simulink model "MotorCtrl_DTC_Math"  (R2023b)
settings: Solver=FixedStepDiscrete  StartTime=0.0  StopTime=5  FixedStep=MC_Sim_BaseStep  RelTol=1e-3  EnableMultiTasking=on
values from neighbouring files (symbols this model uses):
  MC_ADC_BitNum = 0.0    [MotorControlDataDictionary_Math.sldd]
  MC_ADC_Offset = 0.0    [MotorControlDataDictionary_Math.sldd]
  MC_ADC_VRef = 1.0    [MotorControlDataDictionary_Math.sldd]
  MC_Const_DutyL = 0.2    [MotorControlDataDictionary_Math.sldd]
  MC_Const_DutyS = 0.8    [MotorControlDataDictionary_Math.sldd]
  MC_CSA_Gain = 1.0    [MotorControlDataDictionary_Math.sldd]
  MC_Input_Vdc = 13.5    [MotorControlDataDictionary_Math.sldd]
  MC_MOS_DeadTime = 1.0E-6    [MotorControlDataDictionary_Math.sldd]
  MC_Motor_Mechinal_Damp = 1.0E-5    [MotorControlDataDictionary_Math.sldd]
  MC_Motor_Mechinal_Fric = 0.0    [MotorControlDataDictionary_Math.sldd]
  MC_Motor_Mechinal_Inertia = 0.0103    [MotorControlDataDictionary_Math.sldd]
  MC_Motor_Phi = 0.0059190254913385806    [MotorControlDataDictionary_Math.sldd]
  MC_Motor_Rotor_Pn = 4.0    [MotorControlDataDictionary_Math.sldd]
  MC_Motor_Stator_Ld = 5.6345E-5    [MotorControlDataDictionary_Math.sldd]
  MC_Motor_Stator_Lq = 5.6345E-5    [MotorControlDataDictionary_Math.sldd]
  MC_Motor_Stator_Rs = 0.0286    [MotorControlDataDictionary_Math.sldd]
  MC_Param_CurrentPI_Ki = 0.0071879639914134473    [MotorControlDataDictionary_Math.sldd]
  MC_Param_CurrentPI_Kp = 0.283220860906427    [MotorControlDataDictionary_Math.sldd]
  MC_Param_CurrentPI_UdInteMax = 7.794228634059948    [MotorControlDataDictionary_Math.sldd]
  MC_Param_CurrentPI_UdInteMin = -7.794228634059948    [MotorControlDataDictionary_Math.sldd]
  MC_Param_CurrentPI_UdMax = 7.794228634059948    [MotorControlDataDictionary_Math.sldd]
  MC_Param_CurrentPI_UdMin = -7.794228634059948    [MotorControlDataDictionary_Math.sldd]
  MC_Param_CurrentPI_UqInteMax = 7.794228634059948    [MotorControlDataDictionary_Math.sldd]
  MC_Param_CurrentPI_UqInteMin = -7.794228634059948    [MotorControlDataDictionary_Math.sldd]
  MC_Param_CurrentPI_UqMax = 7.794228634059948    [MotorControlDataDictionary_Math.sldd]
  MC_Param_CurrentPI_UqMin = -7.794228634059948    [MotorControlDataDictionary_Math.sldd]
  MC_Param_Flux_Gamma = 750000.0    [MotorControlDataDictionary_Math.sldd]
  MC_Param_Flux_Lalpha = 5.6345E-5    [MotorControlDataDictionary_Math.sldd]
  MC_Param_Flux_Lbeta = 5.6345E-5    [MotorControlDataDictionary_Math.sldd]
  MC_Param_Flux_Ralpha = 0.0286    [MotorControlDataDictionary_Math.sldd]
  MC_Param_Flux_Rbeta = 0.0286    [MotorControlDataDictionary_Math.sldd]
  MC_Param_Luen_BEMFalpha = -17747.803709290976    [MotorControlDataDictionary_Math.sldd]
  MC_Param_Luen_BEMFbeta = -17747.803709290976    [MotorControlDataDictionary_Math.sldd]
  MC_Param_Luen_BEMFErr = -8.0    [MotorControlDataDictionary_Math.sldd]
  MC_Param_Luen_Currentalpha = -507.58718608572195    [MotorControlDataDictionary_Math.sldd]
  MC_Param_Luen_Currentbeta = -507.58718608572195    [MotorControlDataDictionary_Math.sldd]
  MC_Param_Luen_CurrentErr = -8.0    [MotorControlDataDictionary_Math.sldd]
  MC_Param_Luen_PLL_Ki = 2.3480975196640594    [MotorControlDataDictionary_Math.sldd]
  MC_Param_Luen_PLL_Kp = 153.24842212633141    [MotorControlDataDictionary_Math.sldd]
  MC_Param_Luen_Voltagealpha = 17747.803709290976    [MotorControlDataDictionary_Math.sldd]
  MC_Param_Luen_Voltagebeta = 17747.803709290976    [MotorControlDataDictionary_Math.sldd]
  MC_Param_PhasetoReal = 500.0    [MotorControlDataDictionary_Math.sldd]
  MC_Param_SMO_CoffA = 0.97462064069571386    [MotorControlDataDictionary_Math.sldd]
  MC_Param_SMO_CoffB = 0.88739018546454884    [MotorControlDataDictionary_Math.sldd]
  MC_Param_SpeedCtrl_IdMax = 60.0    [MotorControlDataDictionary_Math.sldd]
  MC_Param_SpeedCtrl_IdMin = -60.0    [MotorControlDataDictionary_Math.sldd]
  MC_Param_SpeedCtrl_IqMax = 60.0    [MotorControlDataDictionary_Math.sldd]
  MC_Param_SpeedCtrl_IqMin = -60.0    [MotorControlDataDictionary_Math.sldd]
  MC_Param_SpeedPI_Ki = 0.57248683633241571    [MotorControlDataDictionary_Math.sldd]
  MC_Param_SpeedPI_Kp = 9.1114109857344836    [MotorControlDataDictionary_Math.sldd]
  MC_Param_SpeedtoTheta = 5.0E-5    [MotorControlDataDictionary_Math.sldd]
  MC_Param_SVPWM_DutyMax = 0.98    [MotorControlDataDictionary_Math.sldd]
  MC_Param_SVPWM_DutyMin = 0.02    [MotorControlDataDictionary_Math.sldd]
  MC_Param_SVPWM_SampleOffset1 = 0.02    [MotorControlDataDictionary_Math.sldd]
  MC_Param_SVPWM_SampleOffset2 = 0.015    [MotorControlDataDictionary_Math.sldd]
  MC_Param_SVPWM_SampleValid = 0.011999999999999999    [MotorControlDataDictionary_Math.sldd]
  MC_Sample_CurrentNoise = 1.0E-15    [MotorControlDataDictionary_Math.sldd]
  MC_Sample_Rs = 0.002    [MotorControlDataDictionary_Math.sldd]
  MC_Sample_VbusNoise = 1.0E-15    [MotorControlDataDictionary_Math.sldd]
  MC_Sim_BaseStep = 5.0E-8    [MotorControlDataDictionary_Math.sldd]
  MC_Sim_HFTStep = 5.0E-5    [MotorControlDataDictionary_Math.sldd]
  MC_Sim_MFTStep = 0.002    [MotorControlDataDictionary_Math.sldd]
libraries: simulink x29, spsVoltageMeasurementLib x2, spsDCVoltageSourceLib x1, spsGroundLib x1, spsPermanentMagnetSynchronousMachineLib x1, spsSeriesRLCBranchLib x1, spsThreePhaseVIMeasurementLib x1, spsUniversalBridgeLib x1, sps_lib x1
(part 5 of 5)

== system MotorCtrl_DTC_Math/Hardware_Math/currentSample/getCurrentSample_TRS(Three)/getCurrentSampleB ==
  Current : Inport
  Trigger : TriggerPort  TriggerType=falling  VariantControl=(inherit)
  ADCOffset : Constant  Value=0  SampleTime=-1
  ADCQuality : Gain
  Add : Sum
  CSAGain : Gain
  Data Type Conversion3 : DataTypeConversion  OutDataTypeStr=single  SaturateOnIntegerOverflow=off  RndMeth=Floor
  SampleCurrentB : Outport
  wires:
  Current/1 -> CSAGain/1
  Data Type Conversion3/1 -> SampleCurrentB/1  "SampleCurrentB"
  CSAGain/1 -> Add/2
  Add/1 -> ADCQuality/1
  ADCOffset/1 -> Add/1
  ADCQuality/1 -> Data Type Conversion3/1

== system MotorCtrl_DTC_Math/Hardware_Math/currentSample/getCurrentSample_TRS(Three)/getCurrentSampleC ==
  Current : Inport
  Trigger : TriggerPort  TriggerType=falling  VariantControl=(inherit)
  ADCOffset : Constant  Value=0  SampleTime=-1
  ADCQuality : Gain
  Add : Sum
  CSAGain : Gain
  Data Type Conversion3 : DataTypeConversion  OutDataTypeStr=single  SaturateOnIntegerOverflow=off  RndMeth=Floor
  SampleCurrentC : Outport
  wires:
  ADCQuality/1 -> Data Type Conversion3/1
  ADCOffset/1 -> Add/1
  Add/1 -> ADCQuality/1
  CSAGain/1 -> Add/2
  Data Type Conversion3/1 -> SampleCurrentC/1  "SampleCurrentC"
  Current/1 -> CSAGain/1

== system MotorCtrl_DTC_Math/Hardware_Math/currentSample/getCurrentSample_TRS(Two)/getCurrentSample1 ==
  Current : Inport
  Trigger : TriggerPort  VariantControl=(inherit)
  ADCOffset : Constant  Value=0  SampleTime=-1
  ADCQuality : Gain
  Add : Sum
  CSAGain : Gain
  Data Type Conversion3 : DataTypeConversion  OutDataTypeStr=single  SaturateOnIntegerOverflow=off  RndMeth=Floor
  SampleCurrentUp : Outport
  wires:
  ADCQuality/1 -> Data Type Conversion3/1
  ADCOffset/1 -> Add/1
  Add/1 -> ADCQuality/1
  CSAGain/1 -> Add/2
  Data Type Conversion3/1 -> SampleCurrentUp/1  "SampleCurrentUp"
  Current/1 -> CSAGain/1

== system MotorCtrl_DTC_Math/Hardware_Math/currentSample/getCurrentSample_TRS(Two)/getCurrentSample2 ==
  Current : Inport
  Trigger : TriggerPort  TriggerType=falling  VariantControl=(inherit)
  ADCOffset : Constant  Value=0  SampleTime=-1
  ADCQuality : Gain
  Add : Sum
  CSAGain : Gain
  Data Type Conversion3 : DataTypeConversion  OutDataTypeStr=single  SaturateOnIntegerOverflow=off  RndMeth=Floor
  SampleCurrentDown : Outport
  wires:
  Current/1 -> CSAGain/1
  Data Type Conversion3/1 -> SampleCurrentDown/1  "SampleCurrentDown"
  CSAGain/1 -> Add/2
  Add/1 -> ADCQuality/1
  ADCOffset/1 -> Add/1
  ADCQuality/1 -> Data Type Conversion3/1
